simulink model "BKK5"  (Simulink 7.3)
settings: Solver=ode45  StartTime=0.0  StopTime=100  RelTol=1e-7
libraries: simulink x5
settings Model: Creator=Admin  LastModifiedBy=Sainquake
settings DebuggingCC: StrictBusMsg=ErrorLevel1

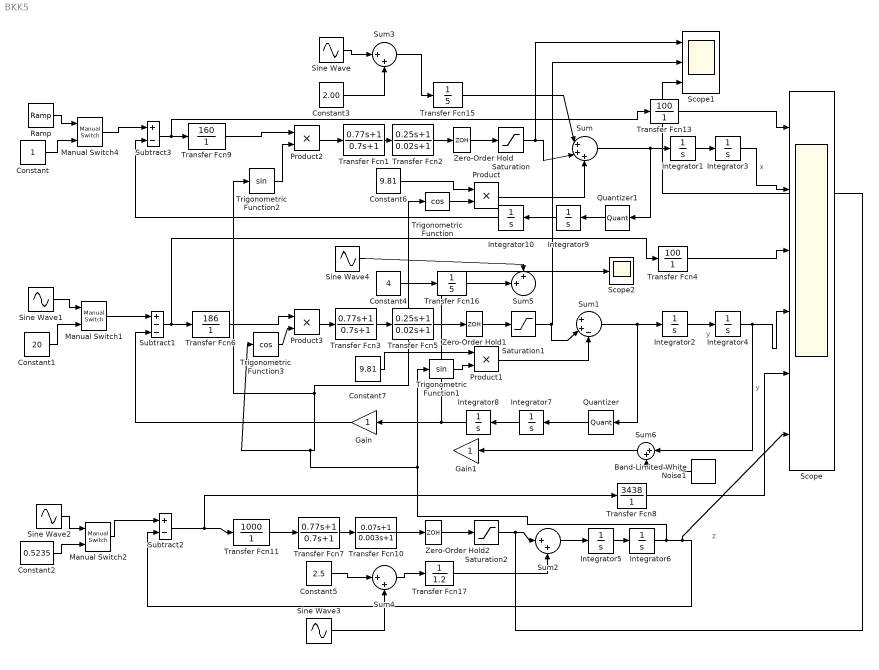
== system BKK5 ==
  note: y
  note: z
  Band-Limited White Noise1 : simulink/Sources/Band-Limited White Noise  SystemSampleTime=-1  Cov=[0.0001]  Ts=1/1000  seed=[23341]
  Constant : Constant
  Constant1 : Constant  Value=20
  Constant2 : Constant  Value=0.5235
  Constant3 : Constant  Value=2.00
  Constant4 : Constant  Value=4
  Constant5 : Constant  Value=2.5
  Constant6 : Constant  Value=9.81
  Constant7 : Constant  Value=9.81
  Gain : Gain  ParameterDataType=fixdt(1, 16)  ParameterScaling=2^0  OutDataType=fixdt(1, 16)  OutScaling=2^0
  Gain1 : Gain  ParameterDataType=fixdt(1, 16)  ParameterScaling=2^0  OutDataType=fixdt(1, 16)  OutScaling=2^0
  Integrator{1..10} (10 alike) : Integrator
  Manual Switch1 : simulink/Signal Routing/Manual Switch  SystemSampleTime=-1  sw=0  action=0  varsize=off
  Manual Switch2 : simulink/Signal Routing/Manual Switch  SystemSampleTime=-1  sw=0  action=0  varsize=off
  Manual Switch4 : simulink/Signal Routing/Manual Switch  SystemSampleTime=-1  sw=0  action=0  varsize=off
  Product{,1..3} (4 alike) : Product  RndMeth=Zero
  Quantizer : Quantizer  QuantizationInterval=0.00390625  SampleTime=1/200
  Quantizer1 : Quantizer  QuantizationInterval=0.00390625  SampleTime=1/200
  Ramp : simulink/Sources/Ramp  SystemSampleTime=-1  slope=1  start=0  X0=0
  Saturation : Saturate  UpperLimit=10  LowerLimit=-10
  Saturation1 : Saturate  UpperLimit=17.2  LowerLimit=-17.2
  Saturation2 : Saturate  UpperLimit=20  LowerLimit=-20
  Scope : Scope  NumInputPorts=6
      settings: YMin=-45~0~-500~0~-750~0  YMax=5~60~2000~25~2000~0.7  MaxDataPoints=5000000
  Scope1 : Scope  NumInputPorts=3
      settings: YMin=-5~-5~-5  YMax=5~5~5  MaxDataPoints=5000000
  Scope2 : Scope
      settings: YMin=4.916  YMax=4.927  SaveName=ScopeData2  MaxDataPoints=500000
  Sine Wave : Sin  Amplitude=0.4  Bias=0  Frequency=0.314  Phase=0  Samples=10  SampleTime=0  Offset=0
  Sine Wave1 : Sin  Amplitude=0.1  Bias=0  Frequency=0.628  Phase=0  Samples=10  SampleTime=0  Offset=0
  Sine Wave2 : Sin  Amplitude=0.1  Bias=0  Frequency=0.628  Phase=0  Samples=10  SampleTime=0  Offset=0
  Sine Wave3 : Sin  Amplitude=0.5  Bias=0  Frequency=6.28  Phase=1.57  Samples=10  SampleTime=0  Offset=0
  Sine Wave4 : Sin  Amplitude=0.3  Bias=0  Frequency=0.3  Phase=1.57  Samples=10  SampleTime=0  Offset=0
  Subtract1 : Sum  Inputs=+--
  Subtract2 : Sum  Inputs=+-
  Subtract3 : Sum  Inputs=+-
  Sum : Sum  Inputs=|+++
  Sum1 : Sum  Inputs=|++-
  Sum2 : Sum  Inputs=|++
  Sum3 : Sum  Inputs=|++
  Sum4 : Sum  Inputs=|++
  Sum5 : Sum  Inputs=++|
  Sum6 : Sum  Inputs=|++  OutDataType=fixdt(1, 16)  OutScaling=2^0
  Transfer Fcn1 : TransferFcn  Numerator=[0.77 1]  Denominator="[0.7  1]"
  Transfer Fcn10 : TransferFcn  Numerator=[0.07 1]  Denominator="[0.003  1]"
  Transfer Fcn11 : TransferFcn  Numerator=1000  Denominator=[ 1 ]
  Transfer Fcn13 : TransferFcn  Numerator=[100]  Denominator=[ 1 ]
  Transfer Fcn15 : TransferFcn  Denominator=[ 5 ]
  Transfer Fcn16 : TransferFcn  Denominator=[ 5 ]
  Transfer Fcn17 : TransferFcn  Denominator=[ 1.2 ]
  Transfer Fcn2 : TransferFcn  Numerator=[0.25 1]  Denominator="[0.02  1]"
  Transfer Fcn3 : TransferFcn  Numerator=[0.77 1]  Denominator="[0.7  1]"
  Transfer Fcn4 : TransferFcn  Numerator=[100]  Denominator=[ 1 ]
  Transfer Fcn5 : TransferFcn  Numerator=[0.25 1]  Denominator="[0.02  1]"
  Transfer Fcn6 : TransferFcn  Numerator=186  Denominator=[ 1 ]
  Transfer Fcn7 : TransferFcn  Numerator=[0.77 1]  Denominator="[0.7  1]"
  Transfer Fcn8 : TransferFcn  Numerator=[3438]  Denominator=[ 1 ]
  Transfer Fcn9 : TransferFcn  Numerator=160  Denominator=[ 1 ]
  Trigonometric Function : Trigonometry  Operator=cos
  Trigonometric Function1 : Trigonometry
  Trigonometric Function2 : Trigonometry
  Trigonometric Function3 : Trigonometry  Operator=cos
  Zero-Order Hold : ZeroOrderHold  SampleTime=0.02
  Zero-Order Hold1 : ZeroOrderHold  SampleTime=1/200
  Zero-Order Hold2 : ZeroOrderHold  SampleTime=1/50
  wires:
  Subtract3/1 -> Transfer Fcn9/1, Transfer Fcn13/1
  Transfer Fcn1/1 -> Transfer Fcn2/1
  Integrator1/1 -> Integrator3/1
  Manual Switch4/1 -> Subtract3/1
  Constant/1 -> Manual Switch4/2
  Transfer Fcn13/1 -> Scope/1
  Subtract1/1 -> Transfer Fcn6/1, Transfer Fcn4/1
  Transfer Fcn3/1 -> Transfer Fcn5/1
  Integrator2/1 -> Integrator4/1
  Transfer Fcn4/1 -> Scope/3
  Subtract2/1 -> Transfer Fcn11/1, Transfer Fcn8/1
  Transfer Fcn11/1 -> Transfer Fcn7/1
  Transfer Fcn7/1 -> Transfer Fcn10/1
  Integrator5/1 -> Integrator6/1
  Integrator6/1 -> Subtract2/2, Scope/6, Trigonometric Function1/1, Trigonometric Function2/1, Trigonometric Function/1, Trigonometric Function3/1
  Transfer Fcn8/1 -> Scope/5
  Constant2/1 -> Manual Switch2/2
  Sine Wave2/1 -> Manual Switch2/1
  Constant1/1 -> Manual Switch1/2
  Integrator3/1 -> Scope/2  "x"
  Integrator4/1 -> Scope/4, Sum6/1  "y"
  Product1/1 -> Sum1/3
  Sum/1 -> Integrator1/1, Quantizer1/1
  Sum1/1 -> Integrator2/1, Quantizer/1
  Transfer Fcn5/1 -> Zero-Order Hold1/1
  Transfer Fcn2/1 -> Zero-Order Hold/1
  Constant4/1 -> Transfer Fcn16/1
  Sum2/1 -> Integrator5/1
  Transfer Fcn10/1 -> Zero-Order Hold2/1
  Transfer Fcn17/1 -> Sum2/2
  Ramp/1 -> Manual Switch4/1
  Sine Wave1/1 -> Manual Switch1/1
  Manual Switch2/1 -> Subtract2/1
  Trigonometric Function/1 -> Product/2
  Constant6/1 -> Product/1
  Trigonometric Function1/1 -> Product1/2
  Constant7/1 -> Product1/1
  Trigonometric Function2/1 -> Product2/2
  Product2/1 -> Transfer Fcn1/1
  Transfer Fcn9/1 -> Product2/1
  Trigonometric Function3/1 -> Product3/2
  Product3/1 -> Transfer Fcn3/1
  Transfer Fcn6/1 -> Product3/1
  Transfer Fcn15/1 -> Sum/1
  Product/1 -> Sum/3
  Sine Wave/1 -> Sum3/1
  Constant3/1 -> Sum3/2
  Sum3/1 -> Transfer Fcn15/1
  Sum4/1 -> Transfer Fcn17/1
  Constant5/1 -> Sum4/1
  Sine Wave3/1 -> Sum4/2
  Zero-Order Hold2/1 -> Saturation2/1
  Zero-Order Hold1/1 -> Saturation1/1
  Zero-Order Hold/1 -> Saturation/1
  Saturation1/1 -> Scope1/2, Sum1/2
  Saturation/1 -> Sum/2, Scope1/1
  Saturation2/1 -> Sum2/1, Scope1/3
  Transfer Fcn16/1 -> Sum5/2
  Sine Wave4/1 -> Sum5/1
  Quantizer/1 -> Integrator7/1
  Band-Limited White Noise1/1 -> Sum6/2
  Gain/1 -> Subtract1/3
  Sum6/1 -> Gain1/1
  Integrator7/1 -> Integrator8/1
  Manual Switch1/1 -> Subtract1/1
  Integrator8/1 -> Gain/1, Scope2/1
  Quantizer1/1 -> Integrator9/1
  Integrator9/1 -> Integrator10/1
  Integrator10/1 -> Subtract3/2
